simulink model "W2P1"  (R2020b)
settings: Solver=VariableStepAuto  StartTime=0.0  StopTime=10.0  RelTol=1e-3
settings Model: Creator=saadh  LastModifiedBy=saadh

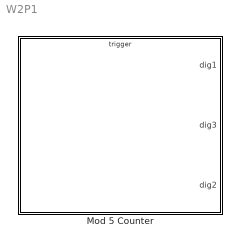
== system W2P1 ==
  Mod 5 Counter : Stateflow chart  TreatAsAtomicUnit=on

== stateflow chart W2P1/Mod 5 Counter ==
  state digit_2 [parallel]
    settings: executionOrder=1
    state two
      en:
      dig2=2;
    state three
      en:
      dig2=3;
    state one
      en:
      dig2=1;
    state Zero
      en:
      dig2=0;
    state four
      en:
      dig2=4;
    digit_2.one -> digit_2.two : input_click2
    digit_2.two -> digit_2.three : input_click2
    digit_2.Zero -> digit_2.one : input_click2
    digit_2.three -> digit_2.four : input_click2
    digit_2.four -> digit_2.Zero : input_click2/{input_click3}
    (default) -> digit_2.Zero
  state digit_1 [parallel]
    settings: executionOrder=2
    state two
      en:
      dig1=2;
    state one
      en:
      dig1=1;
    state three
      en:
      dig1=3;
    state Zero
      en:
      dig1=0
    state four
      en:
      dig1=4;
    digit_1.one -> digit_1.two : input_click
    digit_1.two -> digit_1.three : input_click
    digit_1.Zero -> digit_1.one : input_click
    digit_1.three -> digit_1.four : input_click
    digit_1.four -> digit_1.Zero : input_click/{input_click2}
    (default) -> digit_1.Zero
  state digit_3 [parallel]
    settings: executionOrder=3
    state two
      en:
      dig3=2;
    state one
      en:
      dig3=1;
    state three
      en:
      dig3=3;
    state Zero
      en:
      dig3=0;
    state four
      en:
      dig3=4;
    digit_3.one -> digit_3.two : input_click3
    digit_3.two -> digit_3.three : input_click3
    digit_3.Zero -> digit_3.one : input_click3
    digit_3.three -> digit_3.four : input_click3
    digit_3.four -> digit_3.Zero : input_click3
    (default) -> digit_3.Zero
  data: dig1 output; dig3 output; dig2 output
  events: input_click input FUNCTION_CALL_EVENT; input_click2 local RISING_EDGE_EVENT; input_click3 local RISING_EDGE_EVENT
